simulink model "Third_Harmonic_Injection_Inverter"  (R2015a)
settings: Solver=ode45  StartTime=0.0  StopTime=2  RelTol=1e-3
libraries: powerlib x17, simulink x1
settings Model: Creator=Koustubh  LastModifiedBy=Koustubh

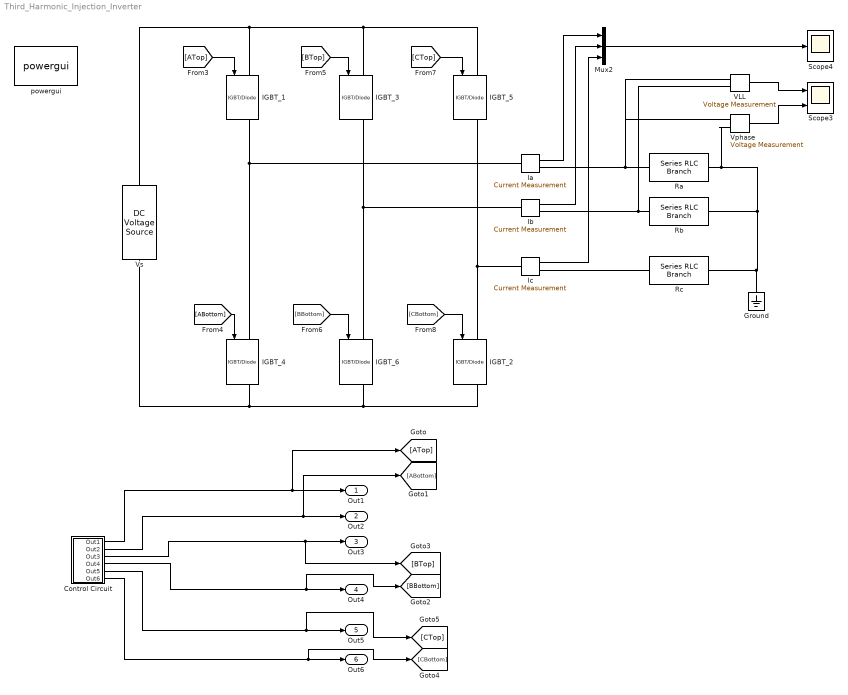
== system Third_Harmonic_Injection_Inverter ==
  Control Circuit : Subsystem
  Ground : powerlib/Elements/Ground  LConnTagsString=a
  IGBT_{1..6} (6 alike) : powerlib/Power Electronics/IGBT//Diode  Ron=1e-3  Rs=1e5  Cs=inf  Measurements=on
  Ia : powerlib/Measurements/Current Measurement  PhasorSimulation=off  OutputType=Complex  PSBequivalent=0
  Ib : powerlib/Measurements/Current Measurement  PhasorSimulation=off  OutputType=Complex  PSBequivalent=0
  Ic : powerlib/Measurements/Current Measurement  PhasorSimulation=off  OutputType=Complex  PSBequivalent=0
  Mux2 : Mux  Inputs=3
  Ra : powerlib/Elements/Series RLC Branch  LConnTagsString=__new0  RConnTagsString=__new0  BranchType=R  Resistance=10  Inductance=1e-3  SetiL0=off  InitialCurrent=0  Capacitance=1e-6  Setx0=off  InitialVoltage=0  Measurements=None
  Rb : powerlib/Elements/Series RLC Branch  LConnTagsString=__new0  RConnTagsString=__new0  BranchType=R  Resistance=10  Inductance=1e-3  SetiL0=off  InitialCurrent=0  Capacitance=1e-6  Setx0=off  InitialVoltage=0  Measurements=None
  Rc : powerlib/Elements/Series RLC Branch  LConnTagsString=__new0  RConnTagsString=__new0  BranchType=R  Resistance=10  Inductance=1e-3  SetiL0=off  InitialCurrent=0  Capacitance=1e-6  Setx0=off  InitialVoltage=0  Measurements=None
  Scope3 : Scope  NumInputPorts=2
      settings: YMin=-5~-5  YMax=5~5  SaveName=ScopeData2
  Scope4 : Scope
      settings: SaveName=ScopeData3
  VLL : powerlib/Measurements/Voltage Measurement  PhasorSimulation=off  OutputType=Complex  PSBequivalent=0
  Vphase : powerlib/Measurements/Voltage Measurement  PhasorSimulation=off  OutputType=Complex  PSBequivalent=0
  Vs : powerlib/Electrical Sources/DC Voltage Source  Amplitude=230  Measurements=None
  powergui : powerlib/powergui  Priority=1  SimulationMode=Discrete  SolverType=Tustin/Backward Euler (TBE)  SampleTime=50e-6  frequency=60  SPID=off  DisableSnubberDevices=off  DisableRonSwitches=off  DisableVfSwitches=off  SwTol=0  DisplayEquations=off  Interpol=off  methode=off  Ts=100  FunctionMessages=off  echomessages=off  HookPort=off  EnableUseOfTLC=off  x0status=blocks  frequencyindice=0  Pbase=100e6  ErrMax=1e-4  Iterations=50  UnitsV=kV  UnitsW=MW  buscounter=0  RestoreLinks=warning  ResistiveCurrentMeasurement=off  Frange=[0:2:500]  Ylog=off  Xlog=on  ShowGrid=off  save=off  variable=ZData  structure=0  ZoomFFT=off  StartTime=0.0  cycles=1  DisplayStyle=1  fundamental=60  FreqAxis=off  MaxFrequency=1000  frequencyindicesteady=1  RmsSteady=1  display=off
  Out1 : Outport
  Out2 : Outport  Port=2
  Out3 : Outport  Port=3
  Out4 : Outport  Port=4
  Out5 : Outport  Port=5
  Out6 : Outport  Port=6
  wires:
  [ATop] -> IGBT_1/1
  [ABottom] -> IGBT_4/1
  [BBottom] -> IGBT_6/1
  [BTop] -> IGBT_3/1
  [CBottom] -> IGBT_2/1
  [CTop] -> IGBT_5/1
  Mux2/1 -> Scope4/1
  Ia/1 -> Mux2/1
  Ib/1 -> Mux2/2
  Ic/1 -> Mux2/3
  VLL/1 -> Scope3/1
  Vphase/1 -> Scope3/2
  Control Circuit/1(Out1) -> [ATop], Out1/1
  Control Circuit/2(Out2) -> [ABottom], Out2/1
  Control Circuit/3(Out3) -> [BTop], Out3/1
  Control Circuit/4(Out4) -> [BBottom], Out4/1
  Control Circuit/5(Out5) -> [CTop], Out5/1
  Control Circuit/6(Out6) -> [CBottom], Out6/1
  connections:
  IGBT_4/LConn1 -- Ia/LConn1 -- IGBT_1/RConn1
  IGBT_6/LConn1 -- Ib/LConn1 -- IGBT_3/RConn1
  IGBT_2/LConn1 -- Ic/LConn1 -- IGBT_5/RConn1
  IGBT_1/LConn1 -- IGBT_3/LConn1 -- IGBT_5/LConn1 -- Vs/RConn1
  IGBT_4/RConn1 -- Vs/LConn1 -- IGBT_6/RConn1 -- IGBT_2/RConn1
  Ra/RConn1 -- Vphase/LConn2 -- Rb/RConn1 -- Rc/RConn1 -- Ground/LConn1
  Ra/LConn1 -- Ia/RConn1 -- VLL/LConn1 -- Vphase/LConn1
  Ib/RConn1 -- VLL/LConn2 -- Rb/LConn1
  Ic/RConn1 -- Rc/LConn1

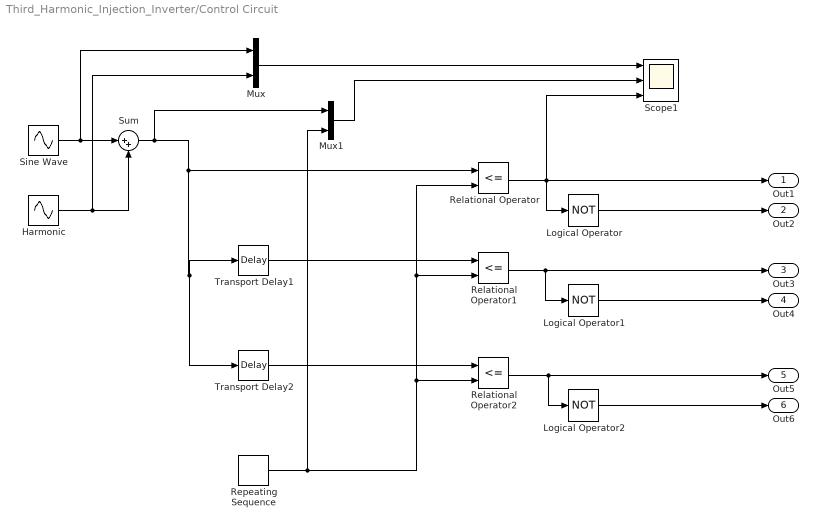
== system Third_Harmonic_Injection_Inverter/Control Circuit ==
  Harmonic : Sin  Amplitude=0.3  Frequency=3*2*pi*50  SampleTime=0
  Logical Operator : Logic  Operator=NOT  AllPortsSameDT=off  OutDataTypeStr=boolean
  Logical Operator1 : Logic  Operator=NOT  AllPortsSameDT=off  OutDataTypeStr=boolean
  Logical Operator2 : Logic  Operator=NOT  AllPortsSameDT=off  OutDataTypeStr=boolean
  Mux : Mux  Inputs=2
  Mux1 : Mux  Inputs=2
  Relational Operator : RelationalOperator  Operator=<=  OutDataTypeStr=boolean
  Relational Operator1 : RelationalOperator  Operator=<=  OutDataTypeStr=boolean
  Relational Operator2 : RelationalOperator  Operator=<=  OutDataTypeStr=boolean
  Repeating Sequence : simulink/Sources/Repeating Sequence  rep_seq_t=[0 0.0005 0.001]  rep_seq_y=[-1 1 -1]
  Scope1 : Scope  NumInputPorts=3
      settings: YMin=-5~-5~-5  YMax=5~5~5
  Sine Wave : Sin  Frequency=2*pi*50  SampleTime=0
  Sum : Sum  Inputs=|++
  Transport Delay1 : TransportDelay  DelayTime=0.006666666667
  Transport Delay2 : TransportDelay  DelayTime=2*0.006666666667
  Out1 : Outport
  Out2 : Outport  Port=2
  Out3 : Outport  Port=3
  Out4 : Outport  Port=4
  Out5 : Outport  Port=5
  Out6 : Outport  Port=6
  wires:
  Mux1/1 -> Scope1/2
  Sum/1 -> Mux1/1, Transport Delay2/1, Transport Delay1/1, Relational Operator/1
  Harmonic/1 -> Mux/2, Sum/2
  Sine Wave/1 -> Mux/1, Sum/1
  Mux/1 -> Scope1/1
  Transport Delay1/1 -> Relational Operator1/1
  Relational Operator2/1 -> Out5/1, Logical Operator2/1
  Logical Operator2/1 -> Out6/1
  Transport Delay2/1 -> Relational Operator2/1
  Repeating Sequence/1 -> Mux1/2, Relational Operator2/2, Relational Operator1/2, Relational Operator/2
  Logical Operator/1 -> Out2/1
  Logical Operator1/1 -> Out4/1
  Relational Operator1/1 -> Out3/1, Logical Operator1/1
  Relational Operator/1 -> Out1/1, Scope1/3, Logical Operator/1
